simulink model "H8_1GDL_2021a"  (R2021b)
settings: Solver=ode4  StartTime=0.0  StopTime=100  FixedStep=1/1000  RelTol=1e-3
InitFcn:
  | m=200;
  | g=9.81;
  | suelo = 0.0225;
  | techo = 0.01;
  | lev_nom = 0.01965;
  | time_stp = 2;
  | %load('force_airgap_current.mat');
  | load('hems.mat');
model workspace (MAT data in the model file):
  surfaceBlockParameters = Simulink.LookupTable
  surfaceBlockParameters.Table = Simulink.lookuptable.Table
  surfaceBlockParameters.Table.Value = [145.669360614  122.326612109  101.996418654  84.6787802495  70.3736968941  59.0811685884  50.8011953324  45.5337771261  43.2789139695  44.0366058625; 185.313749978  156.270189263  130.473313595  107.923122972  88.6196173961  72.5627968658  59.7526613816  50.1892109434  43.8724455513  40.8023652052; 237.482290208  203.298417321  172.595359476  145.373116673  121.631688913  101.371076195  84.59127852  71.2922958872  61.4741282968  55.1367757489; 296.780859506  258.017174483  222.968434498  191.634639553  164.015789646  140.111884779  119.92292495  103.44891016  90.6898404082  81.6457156957; 357.815336073  315.032338952  276.198416866  241.313569815  210.377797799  183.391100818  160.353478873  141.264931963  126.125460088  114.935063248; 415.191598113  368.94978893  326.891184779  289.01578566  255.323591572  225.814602516  200.488818491  179.346239498  162.386865537  149.610696607; 463.515523826  414.37540262  369.652616441  329.347165291  293.459049169  261.988268074  234.934822007  212.298710969  194.079934958  180.278493975; 497.392991416  445.915058223  399.088590054  356.91358691  319.39004879  286.517975694  258.297367623  234.728224576  215.810546553  201.544333555; 511.429879083  458.174633941  409.804983819  366.320928719  327.722468638  294.009603579  265.18233354  241.240658522  222.184578525  208.014093548]
  surfaceBlockParameters.Table.Dimensions = [9 10]
  surfaceBlockParameters.Table.DataType = 'auto'
  surfaceBlockParameters.Table.FieldName = 'Table_force'
  surfaceBlockParameters.Breakpoints(1) = Simulink.lookuptable.Breakpoint
  surfaceBlockParameters.Breakpoints(1).Value = [-40 -31.1 -22.2 -13.3 -4.4 4.5 13.4 22.3 31.2]
  surfaceBlockParameters.Breakpoints(1).TunableSizeName = 'N1'
  surfaceBlockParameters.Breakpoints(1).Dimensions = [1 9]
  surfaceBlockParameters.Breakpoints(1).DataType = 'auto'
  surfaceBlockParameters.Breakpoints(1).FieldName = 'BP1_current'
  surfaceBlockParameters.Breakpoints(2) = Simulink.lookuptable.Breakpoint
  surfaceBlockParameters.Breakpoints(2).Value = [0.011 0.0123 0.0136 0.0149 0.0162 0.0175 0.0188 0.0201 0.0214 0.0227]
  surfaceBlockParameters.Breakpoints(2).TunableSizeName = 'N2'
  surfaceBlockParameters.Breakpoints(2).Dimensions = [1 10]
  surfaceBlockParameters.Breakpoints(2).DataType = 'auto'
  surfaceBlockParameters.Breakpoints(2).FieldName = 'BP2_airgap'
  surfaceBlockParameters.SupportTunableSize = 0
  surfaceBlockParameters.StructTypeInfo = Simulink.lookuptable.StructTypeInfo
  surfaceBlockParameters.StructTypeInfo.Name = 'surfaceBlockParameters_type'
  surfaceBlockParameters.StructTypeInfo.DataScope = 'Auto'
undefined symbols (not defined in the file or in its folder): hems, magnitude
settings Model: Creator=USUARIO  LastModifiedBy=Hyperloop UPV
settings SolverCC: ConcurrentTasks=on  PositivePriorityOrder=on  AutoInsertRateTranBlk=on
settings OptimizationCC: BlockReduction=off  OptimizeBlockIOStorage=off
settings DebuggingCC: TasksWithSamePriorityMsg=none  UnconnectedInputMsg=none  UnconnectedOutputMsg=none  UnconnectedLineMsg=none
settings ModelReferenceCC: EnableRefExpFcnMdlSchedulingChecks=off
settings RTWCC: Description=Simulink Desktop Real-Time  SystemTargetFile=sldrt.tlc  TemplateMakefile=sldrt.tmf  Toolchain=Simulink Real-Time Toolchain  BuildConfiguration=Faster Runs  RTWCompilerOptimization=on  DLArmComputeVersion=20.02.1
settings CodeAppCC: MaxIdLength=95
settings SimulinkDesktopRealTimeCC: TargetPreCompLibLocation=C:\Program Files\MATLAB\R2021b\toolbox\sldrt\lib\win64

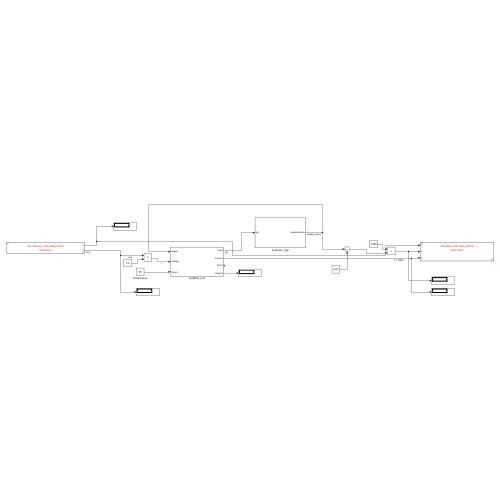
[thumbnail: Simulink's stored preview of the top-level diagram]
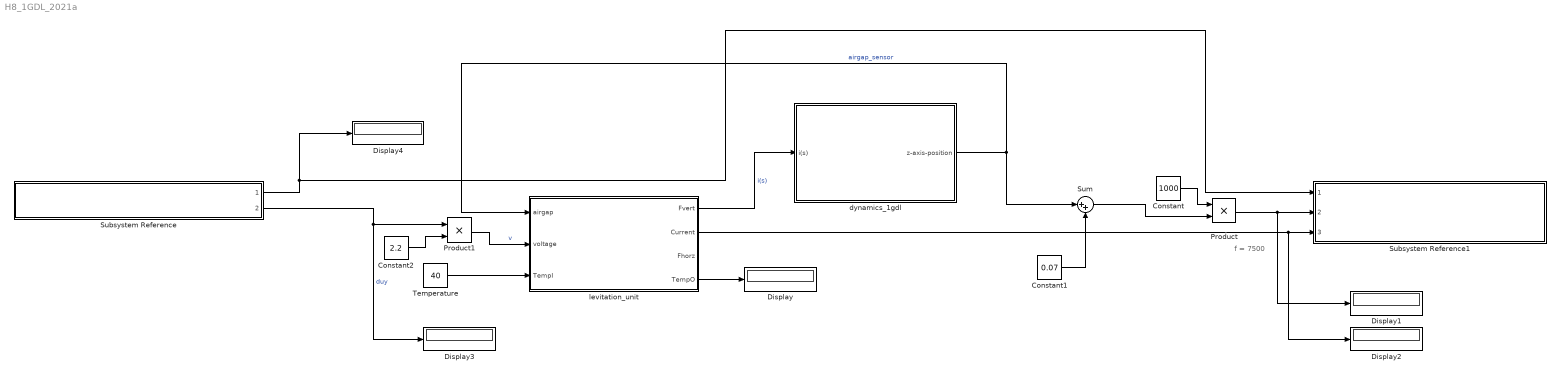
== system H8_1GDL_2021a ==
  note: f = 7500
  Constant : Constant  Value=1000
  Constant1 : Constant  Value=0.07
  Constant2 : Constant  Value=2.2
  Display{,1..4} (5 alike) : Display
  Product : Product
  Product1 : Product
  Subsystem Reference : Subsystem  ReferencedSubsystem=HIL_Receive_TCP_Data_2021a  mi_ip=0  mi_port=0  f=0
  Subsystem Reference1 : Subsystem  ReferencedSubsystem=HIL_Send_TCP_Data_2021a  mi_ip=mi_ip  mi_port=mi_port  f=0
  Sum : Sum  Inputs=|++
  Temperature : Constant  Value=40
  dynamics_1gdl : Subsystem
  levitation_unit : Subsystem
  wires:
  Temperature/1 -> levitation_unit/3(TempI)
  levitation_unit/4(TempO) -> Display/1
  levitation_unit/1(Fvert) -> dynamics_1gdl/1(i(s))  "i(s)"
  dynamics_1gdl/1(z-axis-position) -> Sum/1, levitation_unit/1(airgap)  "airgap_sensor"
  Subsystem Reference/2 -> Display3/1, Product1/1  "duy"
  Subsystem Reference/1 -> Display4/1, Subsystem Reference1/1
  levitation_unit/2(Current) -> Subsystem Reference1/3, Display2/1
  Product/1 -> Subsystem Reference1/2, Display1/1
  Constant/1 -> Product/1
  Sum/1 -> Product/2
  Constant1/1 -> Sum/2
  Product1/1 -> levitation_unit/2(voltage)  "v"
  Constant2/1 -> Product1/2

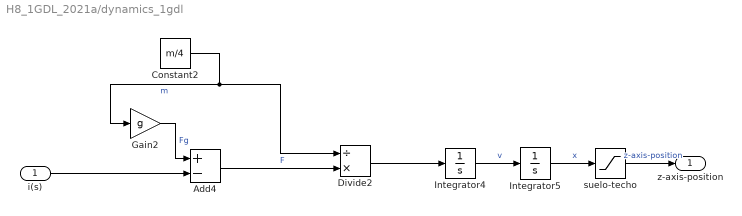
== system H8_1GDL_2021a/dynamics_1gdl ==
  i(s) : Inport
  Add4 : Sum  Inputs=+-
  Constant2 : Constant  Value=m/4
  Divide2 : Product  Inputs=/*
  Gain2 : Gain  Gain=g
  Integrator4 : Integrator
  Integrator5 : Integrator  InitialCondition=suelo  UpperSaturationLimit=suelo
  suelo-techo : Saturate  UpperLimit=suelo  LowerLimit=techo
  z-axis-position : Outport
  wires:
  suelo-techo/1 -> z-axis-position/1  "z-axis-position"
  Constant2/1 -> Divide2/1, Gain2/1  "m"
  Integrator4/1 -> Integrator5/1  "v"
  Add4/1 -> Divide2/2  "F"
  Integrator5/1 -> suelo-techo/1  "x"
  Gain2/1 -> Add4/1  "Fg"
  Divide2/1 -> Integrator4/1
  i(s)/1 -> Add4/2

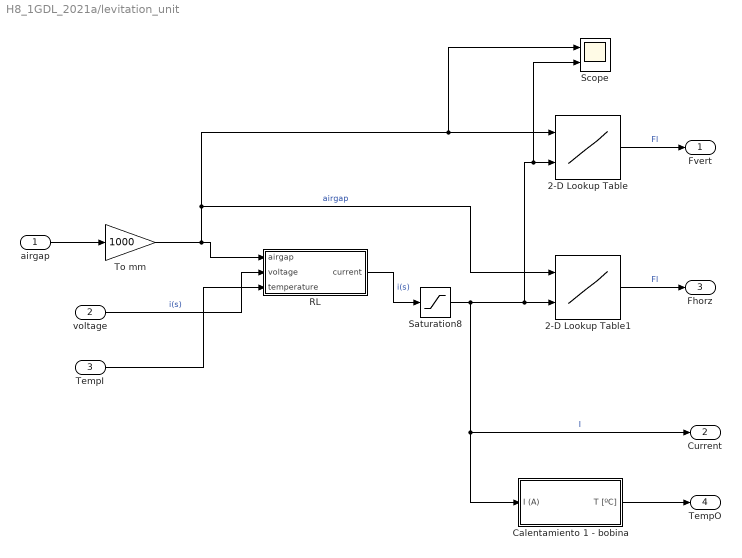
== system H8_1GDL_2021a/levitation_unit ==
  airgap : Inport
  voltage : Inport  Port=2
  TempI : Inport  Port=3
  2-D Lookup Table : Lookup_n-D  BreakpointsForDimension1=hems.Airgap'  BreakpointsForDimension2=hems.Current  Table=hems.Force_Vertical  InternalRulePriority=Speed  RndMeth=Simplest  InputSameDT=on
      settings: InputPortMap=u0,u1
  2-D Lookup Table1 : Lookup_n-D  BreakpointsForDimension1=hems.Airgap'  BreakpointsForDimension2=hems.Current  Table=hems.Force_Horizontal  InternalRulePriority=Speed  RndMeth=Simplest  InputSameDT=on
      settings: InputPortMap=u0,u1
  Calentamiento 1 - bobina : Subsystem
  RL : Subsystem
  Saturation8 : Saturate  UpperLimit=50  LowerLimit=-50
  Scope : Scope  NumInputPorts=2
  To mm : Gain  Gain=1000
  Fvert : Outport
  Current : Outport  Port=2
  Fhorz : Outport  Port=3
  TempO : Outport  Port=4
  wires:
  RL/1(current) -> Saturation8/1  "i(s)"
  voltage/1 -> RL/2(voltage)  "i(s)"
  To mm/1 -> Scope/1, 2-D Lookup Table/1, 2-D Lookup Table1/1, RL/1(airgap)  "airgap"
  Calentamiento 1 - bobina/1(T [ºC]) -> TempO/1
  2-D Lookup Table1/1 -> Fhorz/1  "Fl"
  Saturation8/1 -> Calentamiento 1 - bobina/1(I (A)), Current/1, 2-D Lookup Table1/2, Scope/2, 2-D Lookup Table/2  "I"
  TempI/1 -> RL/3(temperature)
  airgap/1 -> To mm/1
  2-D Lookup Table/1 -> Fvert/1  "Fl"

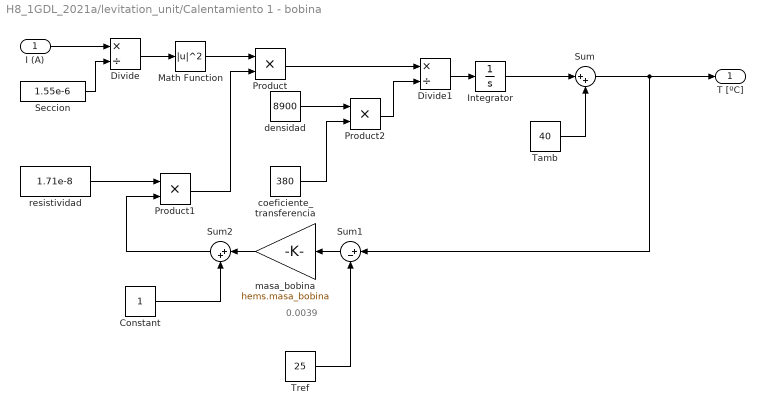
== system H8_1GDL_2021a/levitation_unit/Calentamiento 1 - bobina ==
  note: 0.0039
  I (A) : Inport
  Constant : Constant
  Divide : Product  Inputs=*/
  Divide1 : Product  Inputs=*/
  Integrator : Integrator
  Math Function : Math  Operator=magnitude^2  SaturateOnIntegerOverflow=on
  Product : Product
  Product1 : Product
  Product2 : Product
  Seccion : Constant  Value=1.55e-6
  Sum : Sum  Inputs=|++
  Sum1 : Sum  Inputs=|+-
  Sum2 : Sum  Inputs=|++
  Tamb : Constant  Value=40
  Tref : Constant  Value=25
  coeficiente_transferencia : Constant  Value=380
  densidad : Constant  Value=8900
  masa_bobina : Gain  Gain=hems.masa_bobina
  resistividad : Constant  Value=1.71e-8
  T [ºC] : Outport
  wires:
  I (A)/1 -> Divide/1
  Seccion/1 -> Divide/2
  Divide/1 -> Math Function/1
  Math Function/1 -> Product/1
  Product/1 -> Divide1/1
  Divide1/1 -> Integrator/1
  Integrator/1 -> Sum/1
  Tamb/1 -> Sum/2
  Sum/1 -> Sum1/1, T [ºC]/1
  Sum1/1 -> masa_bobina/1
  Tref/1 -> Sum1/2
  masa_bobina/1 -> Sum2/1
  Constant/1 -> Sum2/2
  resistividad/1 -> Product1/1
  Sum2/1 -> Product1/2
  Product1/1 -> Product/2
  Product2/1 -> Divide1/2
  densidad/1 -> Product2/1
  coeficiente_transferencia/1 -> Product2/2

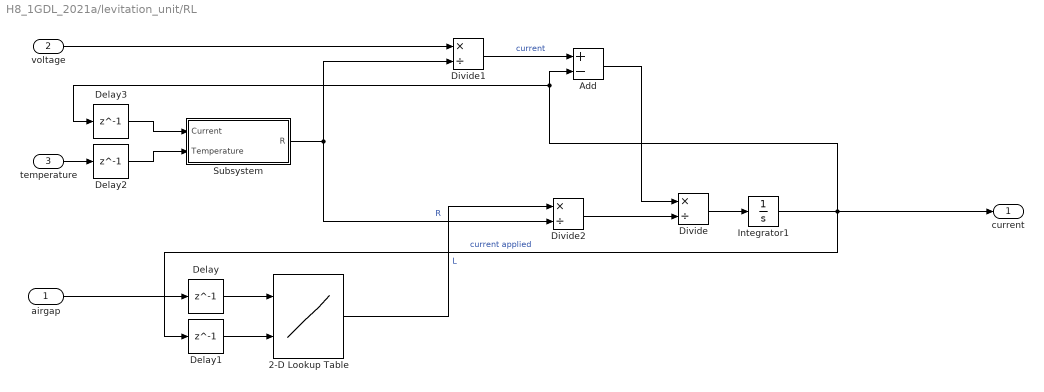
== system H8_1GDL_2021a/levitation_unit/RL ==
  airgap : Inport
  voltage : Inport  Port=2
  temperature : Inport  Port=3
  2-D Lookup Table : Lookup_n-D  BreakpointsForDimension1=hems.Airgap  BreakpointsForDimension2=hems.Current(2:110)  Table=hems.Inductance  InternalRulePriority=Speed  RndMeth=Simplest  InputSameDT=on
      settings: InputPortMap=u0,u1
  Add : Sum  Inputs=+-
  Delay{,1..3} (4 alike) : Delay  DelayLength=1
  Divide : Product  Inputs=*/
  Divide1 : Product  Inputs=*/
  Divide2 : Product  Inputs=*/
  Integrator1 : Integrator
  Subsystem : Subsystem
  current : Outport
  wires:
  airgap/1 -> Delay/1
  Divide/1 -> Integrator1/1
  Add/1 -> Divide/1
  Integrator1/1 -> Delay1/1, current/1, Delay3/1, Add/2  "current applied"
  2-D Lookup Table/1 -> Divide2/1  "L"
  voltage/1 -> Divide1/1
  temperature/1 -> Delay2/1
  Divide1/1 -> Add/1  "current"
  Subsystem/1(R) -> Divide2/2, Divide1/2  "R"
  Delay3/1 -> Subsystem/1(Current)
  Delay2/1 -> Subsystem/2(Temperature)
  Divide2/1 -> Divide/2
  Delay1/1 -> 2-D Lookup Table/2
  Delay/1 -> 2-D Lookup Table/1

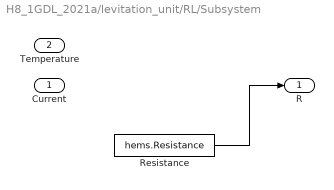
== system H8_1GDL_2021a/levitation_unit/RL/Subsystem ==
  Current : Inport
  Temperature : Inport  Port=2
  Resistance : Constant  Value=hems.Resistance
  R : Outport
  wires:
  Resistance/1 -> R/1
